simulink model "untitled"  (R2021b)
settings: Solver=VariableStepAuto  StartTime=0.0  StopTime=10.0  RelTol=1e-3
libraries: simulink x1
settings Model: Creator=ananagirlea  LastModifiedBy=ananagirlea

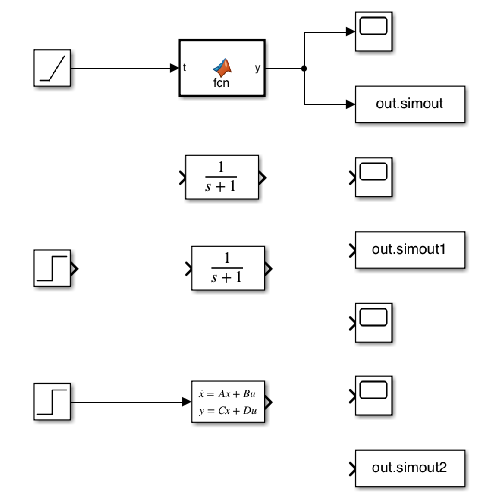
[thumbnail: Simulink's stored preview of the top-level diagram]
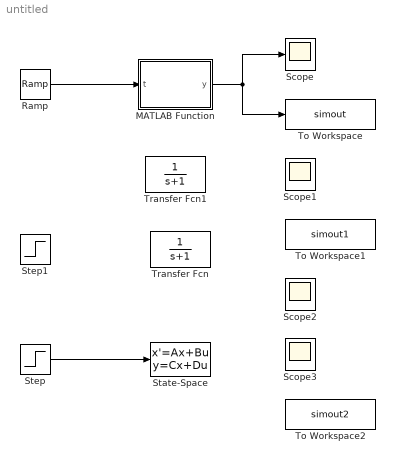
== system untitled ==
  MATLAB Function : MATLAB Function  TreatAsAtomicUnit=on
  Ramp : simulink/Sources/Ramp  slope=1  start=0  InitialOutput=0
  Scope{,1..3} (4 alike) : Scope
  State-Space : StateSpace  A=|  B=[0 ,1; 1, -1; 0, 0]  C=[1 ,0, 101]  D=[0, 0]  InitialCondition=0
      | [-1, 0, 0
      | ; -1, -2, -101;1,1, 0]
  Step : Step  Before=-2  SampleTime=0
  Step1 : Step  Before=1  SampleTime=0
  To Workspace : ToWorkspace  VariableName=simout  SaveFormat=Timeseries  SampleTime=-1
  To Workspace1 : ToWorkspace  VariableName=simout1  SaveFormat=Timeseries  SampleTime=-1
  To Workspace2 : ToWorkspace  VariableName=simout2  SaveFormat=Timeseries  SampleTime=-1
  Transfer Fcn : TransferFcn  Denominator=[1 1]
  Transfer Fcn1 : TransferFcn  Denominator=[1 1]
  wires:
  Ramp/1 -> MATLAB Function/1(t)
  MATLAB Function/1(y) -> Scope/1, To Workspace/1
  Step/1 -> State-Space/1

== matlab function untitled/MATLAB Function ==
  data: t input; y output
function y = fcn(t)
    y = [exp(-t)
         exp(-t)*(cos(10*t)-sin(10*t)/10)-exp(-t)+(101*sin(10*t)*exp(-t))/10
         (sin(10*t)*exp(-t))/10-exp(-t)*(cos(10*t)+sin(10*t)/10)]
end
